simulink model "Pix_FCC_flash"  (R2019b)
settings: Solver=FixedStepAuto  StartTime=0.0  StopTime=inf  RelTol=1e-3  EnableMultiTasking=on
undefined symbols (not defined in the file or in its folder): dev, FCC_PIX_Data, Main, pwm_output0
libraries: px4lib x14, simulink x10, px4Sensorslib x3
(part 1 of 2)
settings Model: ExtModeTrigDuration=10  Creator=The MathWorks, Inc.  LastModifiedBy=guy-m
settings SolverCC: PositivePriorityOrder=on  AutoInsertRateTranBlk=on
settings OptimizationCC: EnhancedBackFolding=on  PassReuseOutputArgsAs=Individual arguments  MaxStackSize=64  OptimizeBlockOrder=speed  DifferentSizesBufferReuse=on  OptimizationCustomize=off  EfficientTunableParamExpr=on
settings DebuggingCC: InheritedTsInSrcMsg=none  MultiTaskCondExecSysMsg=warning  ParameterTunabilityLossMsg=error
settings HardwareCC: ProdBitPerPointer=32  ProdBitPerSizeT=32  ProdBitPerPtrDiffT=32  ProdLargestAtomicInteger=Long  ProdLargestAtomicFloat=Double  ProdWordSize=32  ProdLongLongMode=on  ProdHWDeviceType=ARM Compatible->ARM Cortex
settings SFSimCC: MATLABDynamicMemAlloc=off  CustomCodeUndefinedFunction=UseInterfaceOnly
settings RTWCC: SystemTargetFile=ert.tlc  HardwareBoard=PX4 Pixhawk Series  TLCOptions="-aInlineSetEventsForThisBaseRateFcn=TLC_FALSE -aSuppressMultiTaskScheduler=TLC_FALSE  -aRateBasedStepFcn=0"  TemplateMakefile=ert_default_tmf  Toolchain=GNU Tools for PX4 Autopilots  IncludeHyperlinkInReport=on  TargetLang=C++
settings CodeAppCC: ForceParamTrailComments=on  IgnoreCustomStorageClasses=off  OperatorAnnotations=on  SimulinkDataObjDesc=on  SFDataObjDesc=on  InsertBlockDesc=on
settings ERTTargetCC: SupportVariableSizeSignals=on

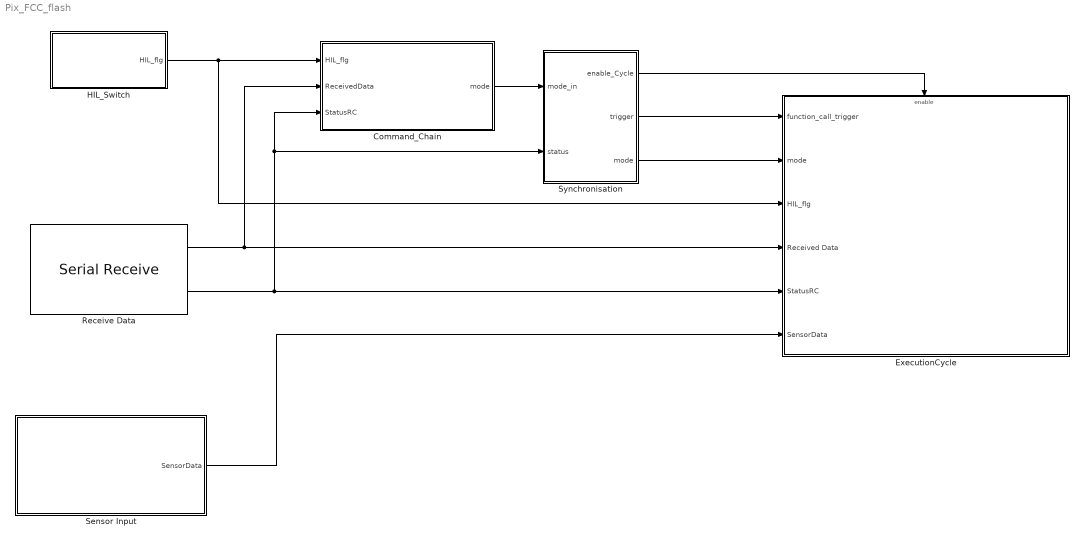
== system Pix_FCC_flash ==
  Command_Chain : Subsystem
  ExecutionCycle : Subsystem
  HIL_Switch : Subsystem
  Receive Data : px4lib/Serial Receive  SCIModule=/dev/ttyS6  DataType=uint8  DataLength=128  OutputStatus=on  SampleTime=0.01  BlockingMode=off  PartialData=off  Timeout=5
      settings: SourceProductName=Embedded Coder Support Package for PX4 Autopilots  SourceProductBaseCode=PX4AUTOPILOTS
  Sensor Input : Subsystem
  Synchronisation : Subsystem
  wires:
  HIL_Switch/1(HIL_flg) -> ExecutionCycle/3(HIL_flg), Command_Chain/1(HIL_flg)
  Command_Chain/1(mode) -> Synchronisation/1(mode_in)
  Synchronisation/1(enable_Cycle) -> ExecutionCycle/Enable
  Synchronisation/2(trigger) -> ExecutionCycle/1(function_call_trigger)
  Receive Data/2 -> ExecutionCycle/5(StatusRC), Command_Chain/3(StatusRC), Synchronisation/2(status)
  Receive Data/1 -> ExecutionCycle/4(Received Data), Command_Chain/2(ReceivedData)
  Synchronisation/3(mode) -> ExecutionCycle/2(mode)
  Sensor Input/1(SensorData) -> ExecutionCycle/6(SensorData)

== system Pix_FCC_flash/Command_Chain ==
  note: sets mode for execution
  note: checks serial input for messages under special command header
  HIL_flg : Inport
  ReceivedData : Inport  Port=2
  StatusRC : Inport  Port=3
  DecodeCommand : Subsystem
  NOT : Logic  Operator=NOT  IconShape=distinctive  AllPortsSameDT=off  OutDataTypeStr=boolean
  SetMode : MATLAB Function  TreatAsAtomicUnit=on
  memory : Subsystem
  mode : Outport  VectorParamsAs1DForOutWhenUnconnected=off
  wires:
  StatusRC/1 -> NOT/1
  ReceivedData/1 -> DecodeCommand/1(message)
  NOT/1 -> DecodeCommand/Enable
  DecodeCommand/2(cmd) -> memory/1(update)
  DecodeCommand/1(cmd_found_flg) -> memory/Enable
  memory/1(standing_cmd) -> SetMode/1(cmd)
  HIL_flg/1 -> SetMode/2(HIL_flg)
  SetMode/1(mode) -> mode/1

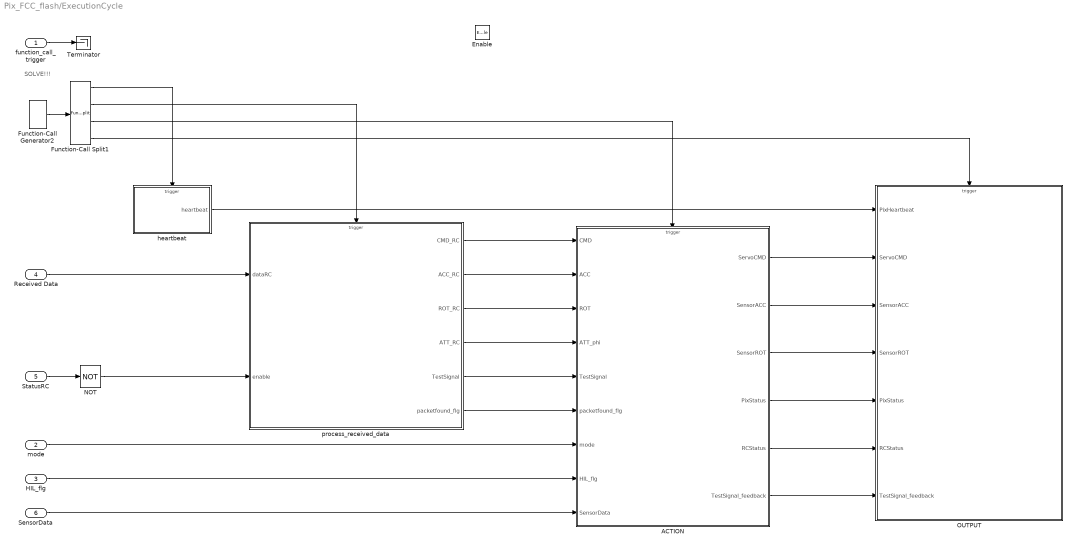
== system Pix_FCC_flash/ExecutionCycle ==
  note: SOLVE!!!
  function_call_trigger : Inport
  mode : Inport  Port=2
  HIL_flg : Inport  Port=3
  Received Data : Inport  Port=4
  StatusRC : Inport  Port=5
  SensorData : Inport  Port=6
  Enable : EnablePort  PropagateVarSize=During execution
  ACTION : Subsystem
  Function-Call Generator2 : simulink/Ports & Subsystems/Function-Call Generator  sample_time=0.01  numberOfIterations=1
  Function-Call Split1 : FunctionCallSplit  IconShape=distinctive  NumOutputPorts=4  OutputPortLayout=default
  NOT : Logic  Operator=NOT  IconShape=distinctive  AllPortsSameDT=off  OutDataTypeStr=boolean
  OUTPUT : Subsystem
  Terminator : Terminator
  heartbeat : Subsystem
  process_received_data : Subsystem
  wires:
  StatusRC/1 -> NOT/1
  NOT/1 -> process_received_data/2(enable)
  Received Data/1 -> process_received_data/1(dataRC)
  process_received_data/1(CMD_RC) -> ACTION/1(CMD)
  process_received_data/2(ACC_RC) -> ACTION/2(ACC)
  process_received_data/3(ROT_RC) -> ACTION/3(ROT)
  process_received_data/4(ATT_RC) -> ACTION/4(ATT_phi)
  process_received_data/6(packetfound_flg) -> ACTION/6(packetfound_flg)
  ACTION/1(ServoCMD) -> OUTPUT/2(ServoCMD)
  ACTION/2(SensorACC) -> OUTPUT/3(SensorACC)
  ACTION/3(SensorROT) -> OUTPUT/4(SensorROT)
  ACTION/4(PixStatus) -> OUTPUT/5(PixStatus)
  heartbeat/1(heartbeat) -> OUTPUT/1(PixHeartbeat)
  Function-Call Split1/1 -> heartbeat/Trigger
  Function-Call Split1/2 -> process_received_data/Trigger
  Function-Call Split1/3 -> ACTION/Trigger
  Function-Call Split1/4 -> OUTPUT/Trigger
  mode/1 -> ACTION/7(mode)
  HIL_flg/1 -> ACTION/8(HIL_flg)
  SensorData/1 -> ACTION/9(SensorData)
  ACTION/5(RCStatus) -> OUTPUT/6(RCStatus)
  process_received_data/5(TestSignal) -> ACTION/5(TestSignal)
  ACTION/6(TestSignal_feedback) -> OUTPUT/7(TestSignal_feedback)
  Function-Call Generator2/1 -> Function-Call Split1/1
  function_call_trigger/1 -> Terminator/1

== system Pix_FCC_flash/HIL_Switch ==
  note: maybe add additional safety? (e.g. for more than one cycle to change?)
  note: in real system this will be done by checking the ADC input for high (HIL connectur plugged in) -> see documentation!!
  Constant : Constant  OutDataTypeStr=boolean
  PX4 Analog Input : px4lib/PX4 Analog Input  Commented=on  sampleTime=0.001
      settings: SourceProductName=Embedded Coder Support Package for PX4 Autopilots  SourceProductBaseCode=PX4AUTOPILOTS
  HIL_flg : Outport  VectorParamsAs1DForOutWhenUnconnected=off
  wires:
  Constant/1 -> HIL_flg/1

== system Pix_FCC_flash/Sensor Input ==
  Accelerometer : px4Sensorslib/Accelerometer  uorbTimeStamp=off  BlockingMode=off  BlockTimeout=1e-3  sampleTime=1/250
      settings: SourceProductName=Embedded Coder Support Package for PX4 Autopilots
  Gyroscope : px4Sensorslib/Gyroscope  uorbTimeStamp=off  BlockingMode=off  BlockTimeout=1e-3  sampleTime=1/250
      settings: SourceProductName=Embedded Coder Support Package for PX4 Autopilots
  Mux : Mux  Inputs=3
  Mux1 : Mux  Inputs=3
  Mux2 : Mux  Inputs=2
  Terminator : Terminator
  Terminator1 : Terminator
  Vehicle Attitude : px4Sensorslib/Vehicle Attitude  rollRate=on  pitchRate=on  yawRate=on  quaternion=on  uorbTimeStamp=off  BlockingMode=off  BlockTimeout=0.001  sampleTime=1/250
      settings: SourceProductName=Embedded Coder Support Package for PX4 Autopilots
  SensorData : Outport  VectorParamsAs1DForOutWhenUnconnected=off
  wires:
  Mux/1 -> Mux2/1
  Mux1/1 -> Mux2/2
  Gyroscope/2 -> Mux1/1
  Accelerometer/1 -> Terminator/1
  Gyroscope/4 -> Mux1/3
  Gyroscope/3 -> Mux1/2
  Accelerometer/3 -> Mux/2
  Accelerometer/4 -> Mux/3
  Accelerometer/2 -> Mux/1
  Gyroscope/1 -> Terminator1/1
  Mux2/1 -> SensorData/1

== system Pix_FCC_flash/Synchronisation ==
  note: SOLVE!!!!
  note: controls the execution of the execution cycle and thereby synchronizes the execution
  mode_in : Inport
  status : Inport  Port=2
  Constant : Constant  Value=0
  ControlExecution : MATLAB Function  TreatAsAtomicUnit=on
  NOT : Logic  Operator=NOT  IconShape=distinctive  AllPortsSameDT=off  OutDataTypeStr=boolean
  trigger_100Hz : Subsystem  Commented=on
  trigger_10Hz : Subsystem  Commented=on
  trigger_inherited : Subsystem  Commented=on
  enable_Cycle : Outport  VectorParamsAs1DForOutWhenUnconnected=off
  trigger : Outport  Port=2  VectorParamsAs1DForOutWhenUnconnected=off
  mode : Outport  Port=3  VectorParamsAs1DForOutWhenUnconnected=off
  wires:
  status/1 -> NOT/1
  mode_in/1 -> mode/1, ControlExecution/1(mode)
  NOT/1 -> ControlExecution/2(status)
  ControlExecution/1(enable_execution) -> enable_Cycle/1
  ControlExecution/2(enable_trigger_inh) -> trigger_inherited/Enable
  ControlExecution/3(enable_trigger_10Hz) -> trigger_10Hz/Enable
  ControlExecution/4(enable_trigger_100Hz) -> trigger_100Hz/Enable
  trigger_inherited/1(trigger) -> ?
  trigger_100Hz/1(trigger) -> ?
  trigger_10Hz/1(trigger) -> ?
  Constant/1 -> trigger/1

== system Pix_FCC_flash/Command_Chain/DecodeCommand ==
  message : Inport
  Enable : EnablePort  PropagateVarSize=During execution
  ConfirmCommand : Subsystem
  DecodeCommand : MATLAB Function  TreatAsAtomicUnit=on
  cmd_found_flg : Outport  VectorParamsAs1DForOutWhenUnconnected=off
  cmd : Outport  Port=2  VectorParamsAs1DForOutWhenUnconnected=off
  wires:
  message/1 -> DecodeCommand/1(message)
  DecodeCommand/2(cmd_found_flg) -> ConfirmCommand/Enable, cmd_found_flg/1
  DecodeCommand/1(cmd) -> ConfirmCommand/1(cmd_received), cmd/1

== system Pix_FCC_flash/Command_Chain/memory ==
  update : Inport
  Enable : EnablePort  PropagateVarSize=During execution
  standing_cmd : Outport  VectorParamsAs1DForOutWhenUnconnected=off
  wires:
  update/1 -> standing_cmd/1

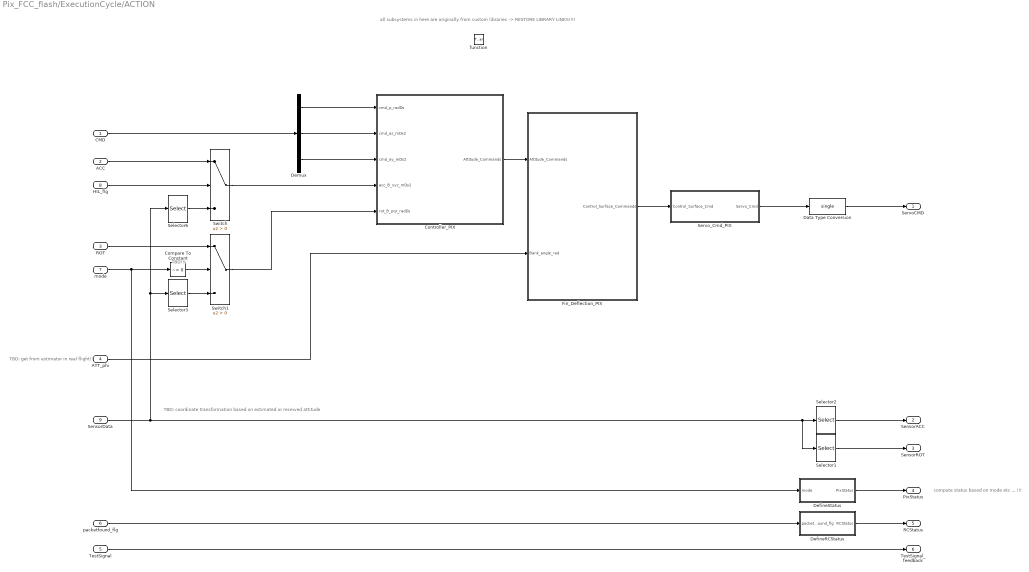
== system Pix_FCC_flash/ExecutionCycle/ACTION ==
  note: TBD: coordinate transformation based on estimated or received attitude
  note: TBD: get from estimator in real flight!!
  note: TBD!!!
  note: compute status based on mode etc ... !!!
  note: all subsystems in here are originally from custom libraries -> RESTORE LIBRARY LINKS!!!!
  CMD : Inport
  ACC : Inport  Port=2
  ROT : Inport  Port=3
  ATT_phi : Inport  Port=4
  TestSignal : Inport  Port=5
  packetfound_flg : Inport  Port=6
  mode : Inport  Port=7
  HIL_flg : Inport  Port=8
  SensorData : Inport  Port=9
  function : TriggerPort  TriggerType=function-call  VariantControl=Variant
  Compare To Constant : simulink/Logic and Bit Operations/Compare To Constant  relop=~=  const=0  OutDataTypeStr=boolean
  Controller_PIX : Subsystem
  Data Type Conversion : DataTypeConversion  OutDataTypeStr=single
  DefineRCStatus : MATLAB Function  TreatAsAtomicUnit=on
  DefineStatus : MATLAB Function  TreatAsAtomicUnit=on
  Demux : Demux  Outputs=3
  Fin_Deflection_PIX : Subsystem
  Selector1 : Selector  InputPortWidth=6  IndexOptions=Index vector (dialog)  Indices=[4,5,6]  OutputSizes=1
  Selector2 : Selector  InputPortWidth=6  IndexOptions=Index vector (dialog)  Indices=[1,2,3]  OutputSizes=1
  Selector3 : Selector  InputPortWidth=6  IndexOptions=Index vector (dialog)  Indices=[4,5,6]  OutputSizes=1
  Selector6 : Selector  InputPortWidth=6  IndexOptions=Index vector (dialog)  Indices=[1,2,3]  OutputSizes=1
  Servo_Cmd_PIX : Subsystem
  Switch : Switch  Criteria=u2 > Threshold
  Switch1 : Switch  Criteria=u2 > Threshold
  ServoCMD : Outport  VectorParamsAs1DForOutWhenUnconnected=off
  SensorACC : Outport  Port=2  VectorParamsAs1DForOutWhenUnconnected=off
  SensorROT : Outport  Port=3  VectorParamsAs1DForOutWhenUnconnected=off
  PixStatus : Outport  Port=4  VectorParamsAs1DForOutWhenUnconnected=off
  RCStatus : Outport  Port=5  VectorParamsAs1DForOutWhenUnconnected=off
  TestSignal_feedback : Outport  Port=6  VectorParamsAs1DForOutWhenUnconnected=off
  wires:
  CMD/1 -> Demux/1
  Servo_Cmd_PIX/1(Servo_Cmd) -> Data Type Conversion/1
  ATT_phi/1 -> Fin_Deflection_PIX/2(Bank_angle_rad)
  Controller_PIX/1(Attitude_Commands) -> Fin_Deflection_PIX/1(Attitude_Commands)
  Fin_Deflection_PIX/1(Control_Surface_Commands) -> Servo_Cmd_PIX/1(Control_Surface_Cmd)
  HIL_flg/1 -> Switch/2
  Switch/1 -> Controller_PIX/4(acc_B_xyz_mDs2)
  Demux/3 -> Controller_PIX/3(cmd_ay_mDs2)
  Demux/2 -> Controller_PIX/2(cmd_az_mDs2)
  Demux/1 -> Controller_PIX/1(cmd_p_radDs)
  Selector2/1 -> SensorACC/1
  Selector1/1 -> SensorROT/1
  ACC/1 -> Switch/1
  Selector6/1 -> Switch/3
  SensorData/1 -> Selector1/1, Selector2/1, Selector3/1, Selector6/1
  Compare To Constant/1 -> Switch1/2
  mode/1 -> DefineStatus/1(mode), Compare To Constant/1
  ROT/1 -> Switch1/1
  Selector3/1 -> Switch1/3
  Switch1/1 -> Controller_PIX/5(rot_B_pqr_radDs)
  packetfound_flg/1 -> DefineRCStatus/1(packetfound_flg)
  DefineStatus/1(PixStatus) -> PixStatus/1
  DefineRCStatus/1(RCStatus) -> RCStatus/1
  TestSignal/1 -> TestSignal_feedback/1
  Data Type Conversion/1 -> ServoCMD/1

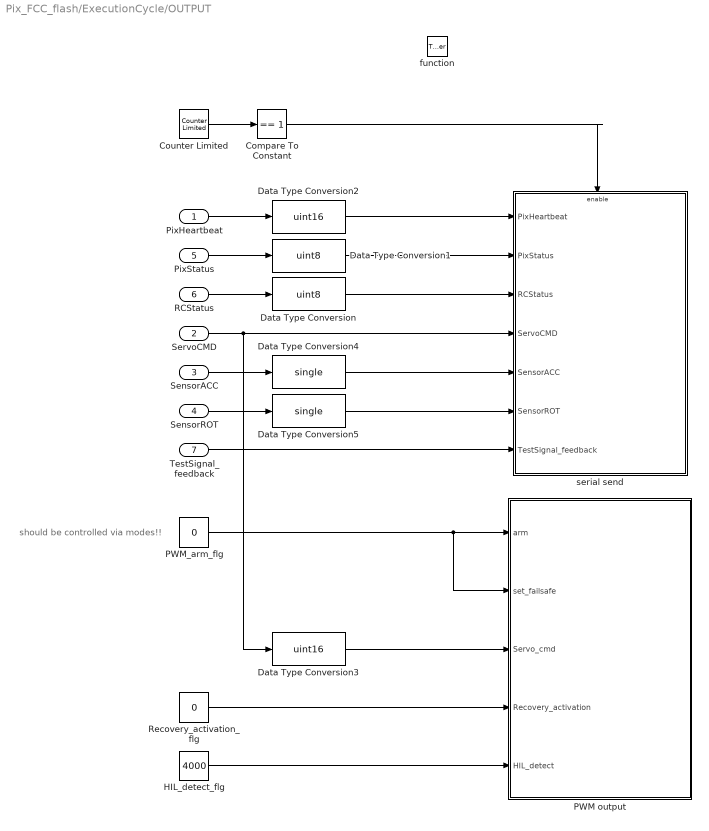
== system Pix_FCC_flash/ExecutionCycle/OUTPUT ==
  note: should be controlled via modes!!
  PixHeartbeat : Inport
  ServoCMD : Inport  Port=2
  SensorACC : Inport  Port=3
  SensorROT : Inport  Port=4
  PixStatus : Inport  Port=5
  RCStatus : Inport  Port=6
  TestSignal_feedback : Inport  Port=7
  function : TriggerPort  TriggerType=function-call  VariantControl=Variant
  Compare To Constant : simulink/Logic and Bit Operations/Compare To Constant  relop===  const=1  OutDataTypeStr=boolean
  Counter Limited : simulink/Sources/Counter Limited  uplimit=1  tsamp=-1
  Data Type Conversion : DataTypeConversion  OutDataTypeStr=uint8
  Data Type Conversion1 : DataTypeConversion  OutDataTypeStr=uint8
  Data Type Conversion2 : DataTypeConversion  OutDataTypeStr=uint16
  Data Type Conversion3 : DataTypeConversion  OutDataTypeStr=uint16
  Data Type Conversion4 : DataTypeConversion  OutDataTypeStr=single
  Data Type Conversion5 : DataTypeConversion  OutDataTypeStr=single
  HIL_detect_flg : Constant  Value=4000  OutDataTypeStr=uint16
  PWM output : Subsystem
  PWM_arm_flg : Constant  Value=0  OutDataTypeStr=boolean
  Recovery_activation_flg : Constant  Value=0  OutDataTypeStr=uint16
  serial send : Subsystem
  wires:
  Counter Limited/1 -> Compare To Constant/1
  Compare To Constant/1 -> serial send/Enable
  PixHeartbeat/1 -> Data Type Conversion2/1
  PixStatus/1 -> Data Type Conversion1/1
  RCStatus/1 -> Data Type Conversion/1
  SensorACC/1 -> Data Type Conversion4/1
  SensorROT/1 -> Data Type Conversion5/1
  Data Type Conversion/1 -> serial send/3(RCStatus)
  Data Type Conversion1/1 -> serial send/2(PixStatus)
  Data Type Conversion2/1 -> serial send/1(PixHeartbeat)
  PWM_arm_flg/1 -> PWM output/2(set_failsafe), PWM output/1(arm)
  HIL_detect_flg/1 -> PWM output/5(HIL_detect)
  Recovery_activation_flg/1 -> PWM output/4(Recovery_activation)
  TestSignal_feedback/1 -> serial send/7(TestSignal_feedback)
  ServoCMD/1 -> serial send/4(ServoCMD), Data Type Conversion3/1
  Data Type Conversion3/1 -> PWM output/3(Servo_cmd)
  Data Type Conversion5/1 -> serial send/6(SensorROT)
  Data Type Conversion4/1 -> serial send/5(SensorACC)

== system Pix_FCC_flash/ExecutionCycle/heartbeat ==
  function : TriggerPort  TriggerType=function-call  VariantControl=Variant
  Add : Sum  Commented=on
  Constant : Constant  Commented=on
  Counter Free-Running : simulink/Sources/Counter Free-Running  NumBits=16  tsamp=-1
  Data Type Conversion1 : DataTypeConversion  Commented=on  OutDataTypeStr=single
  IC : InitialCondition  Commented=on  Value=0
  Memory : Memory  Commented=on  InheritSampleTime=on
  heartbeat : Outport  VectorParamsAs1DForOutWhenUnconnected=off
  wires:
  IC/1 -> Add/2
  Constant/1 -> Add/1
  Add/1 -> Data Type Conversion1/1, Memory/1
  Memory/1 -> IC/1
  Counter Free-Running/1 -> heartbeat/1

== system Pix_FCC_flash/ExecutionCycle/process_received_data ==
  dataRC : Inport
  enable : Inport  Port=2
  function : TriggerPort  TriggerType=function-call  VariantControl=Variant
  Terminator : Terminator
  Terminator1 : Terminator
  Terminator2 : Terminator
  input_hold : Subsystem
  CMD_RC : Outport  VectorParamsAs1DForOutWhenUnconnected=off
  ACC_RC : Outport  Port=2  VectorParamsAs1DForOutWhenUnconnected=off
  ROT_RC : Outport  Port=3  VectorParamsAs1DForOutWhenUnconnected=off
  ATT_RC : Outport  Port=4  VectorParamsAs1DForOutWhenUnconnected=off
  TestSignal : Outport  Port=5  VectorParamsAs1DForOutWhenUnconnected=off
  packetfound_flg : Outport  Port=6  VectorParamsAs1DForOutWhenUnconnected=off
  wires:
  dataRC/1 -> input_hold/1(dataRC)
  input_hold/9(packetfound_flg) -> packetfound_flg/1
  enable/1 -> input_hold/Enable
  input_hold/2(SimStatus) -> Terminator/1
  input_hold/3(SimRCStatus) -> Terminator1/1
  input_hold/1(SimHeartbeat) -> Terminator2/1
  input_hold/4(CMD) -> CMD_RC/1
  input_hold/5(ACC) -> ACC_RC/1
  input_hold/6(ROT) -> ROT_RC/1
  input_hold/7(ATT) -> ATT_RC/1
  input_hold/8(TestSignal) -> TestSignal/1

== system Pix_FCC_flash/Synchronisation/trigger_100Hz ==
  Enable : EnablePort
  Function-Call Generator2 : simulink/Ports & Subsystems/Function-Call Generator  sample_time=0.01  numberOfIterations=1
  trigger : Outport  VectorParamsAs1DForOutWhenUnconnected=off
  wires:
  Function-Call Generator2/1 -> trigger/1

== system Pix_FCC_flash/Synchronisation/trigger_10Hz ==
  Enable : EnablePort
  Function-Call Generator2 : simulink/Ports & Subsystems/Function-Call Generator  sample_time=0.1  numberOfIterations=1
  trigger : Outport  VectorParamsAs1DForOutWhenUnconnected=off
  wires:
  Function-Call Generator2/1 -> trigger/1

== system Pix_FCC_flash/Synchronisation/trigger_inherited ==
  Enable : EnablePort
  Function-Call Generator2 : simulink/Ports & Subsystems/Function-Call Generator  sample_time=-1  numberOfIterations=1
  trigger : Outport  VectorParamsAs1DForOutWhenUnconnected=off
  wires:
  Function-Call Generator2/1 -> trigger/1

== system Pix_FCC_flash/Command_Chain/DecodeCommand/ConfirmCommand ==
  cmd_received : Inport
  Enable : EnablePort  PropagateVarSize=During execution
  Function-Call Generator1 : simulink/Ports & Subsystems/Function-Call Generator  sample_time=-1  numberOfIterations=1
  Function-Call Split : FunctionCallSplit  IconShape=distinctive  NumOutputPorts=6  OutputPortLayout=default
  Send Data : Subsystem
  Send Header : Subsystem  TreatAsAtomicUnit=on
  Send RC Confrimation : Subsystem  TreatAsAtomicUnit=on
  Send Terminator : Subsystem  TreatAsAtomicUnit=on
  Send WhiteNoise Beginning : Subsystem  TreatAsAtomicUnit=on
  Send WhiteNoise End : Subsystem  TreatAsAtomicUnit=on
  pack : MATLAB Function  TreatAsAtomicUnit=on
  wires:
  Function-Call Split/6 -> Send WhiteNoise End/Trigger
  Function-Call Split/5 -> Send Terminator/Trigger
  Function-Call Split/4 -> Send Data/Trigger
  Function-Call Split/1 -> Send WhiteNoise Beginning/Trigger
  pack/1(send) -> Send Data/1(data)
  Function-Call Generator1/1 -> Function-Call Split/1
  Function-Call Split/2 -> Send Header/Trigger
  Function-Call Split/3 -> Send RC Confrimation/Trigger
  cmd_received/1 -> pack/1(in)

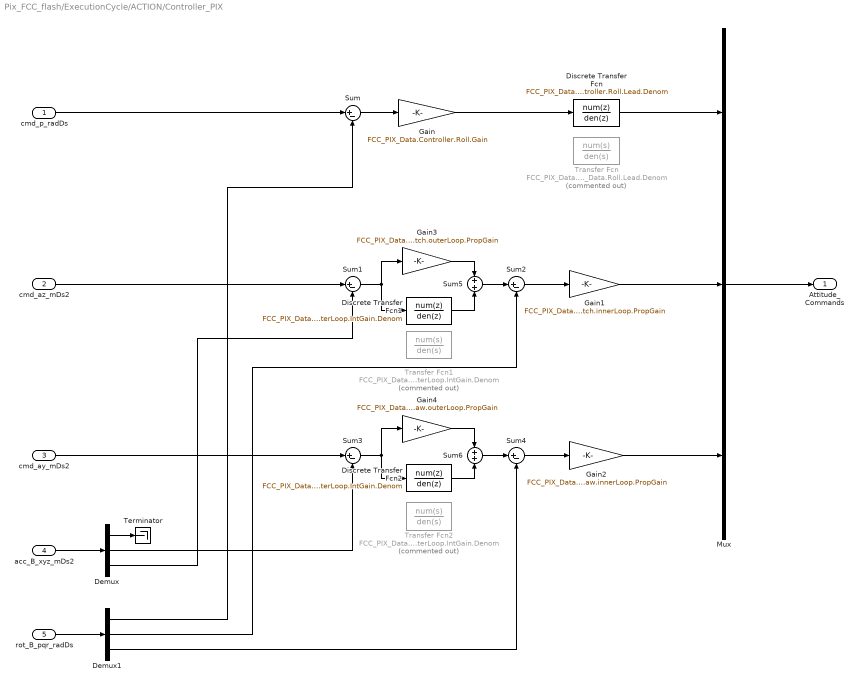
== system Pix_FCC_flash/ExecutionCycle/ACTION/Controller_PIX ==
  cmd_p_radDs : Inport
  cmd_az_mDs2 : Inport  Port=2
  cmd_ay_mDs2 : Inport  Port=3
  acc_B_xyz_mDs2 : Inport  Port=4
  rot_B_pqr_radDs : Inport  Port=5
  Demux : Demux  Outputs=3
  Demux1 : Demux  Outputs=3
  Discrete Transfer Fcn : DiscreteTransferFcn  Numerator=FCC_PIX_Data.Controller.Roll.Lead.Num  Denominator=FCC_PIX_Data.Controller.Roll.Lead.Denom
  Discrete Transfer Fcn1 : DiscreteTransferFcn  Numerator=FCC_PIX_Data.Controller.Pitch.outerLoop.IntGain.Num  Denominator=FCC_PIX_Data.Controller.Pitch.outerLoop.IntGain.Denom
  Discrete Transfer Fcn2 : DiscreteTransferFcn  Numerator=FCC_PIX_Data.Controller.Yaw.outerLoop.IntGain.Num  Denominator=FCC_PIX_Data.Controller.Yaw.outerLoop.IntGain.Denom
  Gain : Gain  Gain=FCC_PIX_Data.Controller.Roll.Gain
  Gain1 : Gain  Gain=FCC_PIX_Data.Controller.Pitch.innerLoop.PropGain
  Gain2 : Gain  Gain=FCC_PIX_Data.Controller.Yaw.innerLoop.PropGain
  Gain3 : Gain  Gain=FCC_PIX_Data.Controller.Pitch.outerLoop.PropGain
  Gain4 : Gain  Gain=FCC_PIX_Data.Controller.Yaw.outerLoop.PropGain
  Mux : Mux  Inputs=3
  Sum{,1..4} (5 alike) : Sum  Inputs=|+-
  Sum5 : Sum  Inputs=+|+
  Sum6 : Sum  Inputs=+|+
  Terminator : Terminator
  Transfer Fcn : TransferFcn  Commented=on  Numerator=FCC_PIX_Data.Roll.Lead.Num  Denominator=FCC_PIX_Data.Roll.Lead.Denom
  Transfer Fcn1 : TransferFcn  Commented=on  Numerator=FCC_PIX_Data.Controller.Pitch.outerLoop.IntGain.Num  Denominator=FCC_PIX_Data.Controller.Pitch.outerLoop.IntGain.Denom
  Transfer Fcn2 : TransferFcn  Commented=on  Numerator=FCC_PIX_Data.Controller.Yaw.outerLoop.IntGain.Num  Denominator=FCC_PIX_Data.Controller.Yaw.outerLoop.IntGain.Denom
  Attitude_Commands : Outport  VectorParamsAs1DForOutWhenUnconnected=off
  wires:
  Demux/1 -> Terminator/1
  Demux/3 -> Sum1/2
  Demux/2 -> Sum3/2
  Demux1/3 -> Sum4/2
  Demux1/2 -> Sum2/2
  Demux1/1 -> Sum/2
  rot_B_pqr_radDs/1 -> Demux1/1
  acc_B_xyz_mDs2/1 -> Demux/1
  Mux/1 -> Attitude_Commands/1
  Discrete Transfer Fcn/1 -> Mux/1
  Gain1/1 -> Mux/2
  Gain2/1 -> Mux/3
  cmd_az_mDs2/1 -> Sum1/1
  cmd_ay_mDs2/1 -> Sum3/1
  cmd_p_radDs/1 -> Sum/1
  Sum3/1 -> Discrete Transfer Fcn2/1, Gain4/1
  Discrete Transfer Fcn2/1 -> Sum6/2
  Gain4/1 -> Sum6/1
  Sum/1 -> Gain/1
  Sum4/1 -> Gain2/1
  Sum2/1 -> Gain1/1
  Gain/1 -> Discrete Transfer Fcn/1
  Sum5/1 -> Sum2/1
  Discrete Transfer Fcn1/1 -> Sum5/2
  Gain3/1 -> Sum5/1
  Sum1/1 -> Discrete Transfer Fcn1/1, Gain3/1
  Sum6/1 -> Sum4/1

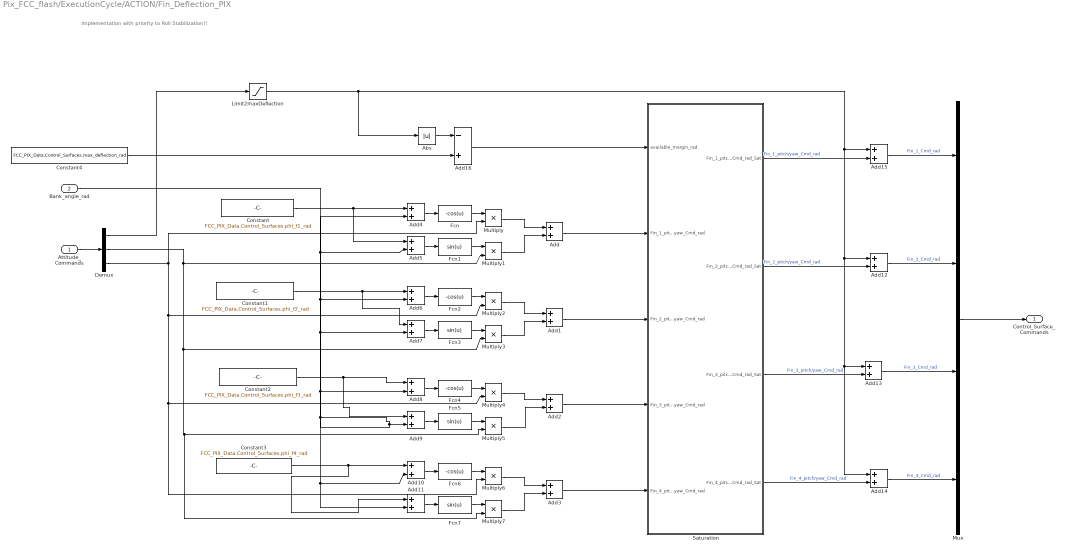
== system Pix_FCC_flash/ExecutionCycle/ACTION/Fin_Deflection_PIX ==
  note: Implementation with priority to Roll Stabilization!!
  Attitude_Commands : Inport
  Bank_angle_rad : Inport  Port=2
  Abs : Abs
  Add{,1..15} (16 alike) : Sum
  Add16 : Sum  Inputs=-+
  Constant : Constant  Value=FCC_PIX_Data.Control_Surfaces.phi_f1_rad
  Constant1 : Constant  Value=FCC_PIX_Data.Control_Surfaces.phi_f2_rad
  Constant2 : Constant  Value=FCC_PIX_Data.Control_Surfaces.phi_f3_rad
  Constant3 : Constant  Value=FCC_PIX_Data.Control_Surfaces.phi_f4_rad
  Constant4 : Constant  Value=FCC_PIX_Data.Control_Surfaces.max_deflection_rad
  Demux : Demux  Outputs=3
  Fcn{,2,4,6} (4 alike) : Fcn  Expr=-cos(u)
  Fcn{1,3,5,7} (4 alike) : Fcn  Expr=sin(u)
  Limit2maxDeflection : Saturate  UpperLimit=FCC_PIX_Data.Control_Surfaces.max_deflection_rad  LowerLimit=-FCC_PIX_Data.Control_Surfaces.max_deflection_rad
  Multiply{,1..7} (8 alike) : Product
  Mux : Mux
  Saturation : Subsystem
  Control_Surface_Commands : Outport  VectorParamsAs1DForOutWhenUnconnected=off
  wires:
  Limit2maxDeflection/1 -> Add15/1, Add12/1, Add13/1, Add14/1, Abs/1
  Saturation/4(Fin_4_pitch/yaw_Cmd_rad_Sat) -> Add14/2  "Fin_4_pitch/yaw_Cmd_rad"
  Saturation/3(Fin_3_pitch/yaw_Cmd_rad_Sat) -> Add13/2  "Fin_3_pitch/yaw_Cmd_rad"
  Saturation/2(Fin_2_pitch/yaw_Cmd_rad_Sat) -> Add12/2  "Fin_2_pitch/yaw_Cmd_rad"
  Saturation/1(Fin_1_pitch/yaw_Cmd_rad_Sat) -> Add15/2  "Fin_1_pitch/yaw_Cmd_rad"
  Add16/1 -> Saturation/1(available_margin_rad)
  Constant4/1 -> Add16/2
  Abs/1 -> Add16/1
  Demux/1 -> Limit2maxDeflection/1
  Add14/1 -> Mux/4  "Fin_4_Cmd_rad"
  Add13/1 -> Mux/3  "Fin_3_Cmd_rad"
  Add12/1 -> Mux/2  "Fin_2_Cmd_rad"
  Add15/1 -> Mux/1  "Fin_1_Cmd_rad"
  Add3/1 -> Saturation/5(Fin_4_pitch/yaw_Cmd_rad)
  Add2/1 -> Saturation/4(Fin_3_pitch/yaw_Cmd_rad)
  Add1/1 -> Saturation/3(Fin_2_pitch/yaw_Cmd_rad)
  Add/1 -> Saturation/2(Fin_1_pitch/yaw_Cmd_rad)
  Mux/1 -> Control_Surface_Commands/1
  Attitude_Commands/1 -> Demux/1
  Constant/1 -> Add4/1, Add5/1
  Constant1/1 -> Add6/1, Add7/1
  Constant2/1 -> Add8/1, Add9/1
  Constant3/1 -> Add10/1, Add11/1
  Bank_angle_rad/1 -> Add9/2, Add8/2, Add6/2, Add5/2, Add4/2, Add7/2, Add10/2, Add11/2
  Multiply7/1 -> Add3/2
  Multiply6/1 -> Add3/1
  Multiply5/1 -> Add2/2
  Multiply4/1 -> Add2/1
  Multiply3/1 -> Add1/2
  Multiply2/1 -> Add1/1
  Multiply1/1 -> Add/2
  Multiply/1 -> Add/1
  Demux/3 -> Multiply2/2, Multiply4/2, Multiply6/2, Multiply/2
  Demux/2 -> Multiply1/2, Multiply3/2, Multiply7/2, Multiply5/2
  Fcn7/1 -> Multiply7/1
  Add10/1 -> Fcn6/1
  Fcn6/1 -> Multiply6/1
  Add11/1 -> Fcn7/1
  Add9/1 -> Fcn5/1
  Fcn4/1 -> Multiply4/1
  Add8/1 -> Fcn4/1
  Fcn5/1 -> Multiply5/1
  Fcn3/1 -> Multiply3/1
  Fcn2/1 -> Multiply2/1
  Add6/1 -> Fcn2/1
  Add7/1 -> Fcn3/1
  Fcn1/1 -> Multiply1/1
  Add5/1 -> Fcn1/1
  Fcn/1 -> Multiply/1
  Add4/1 -> Fcn/1

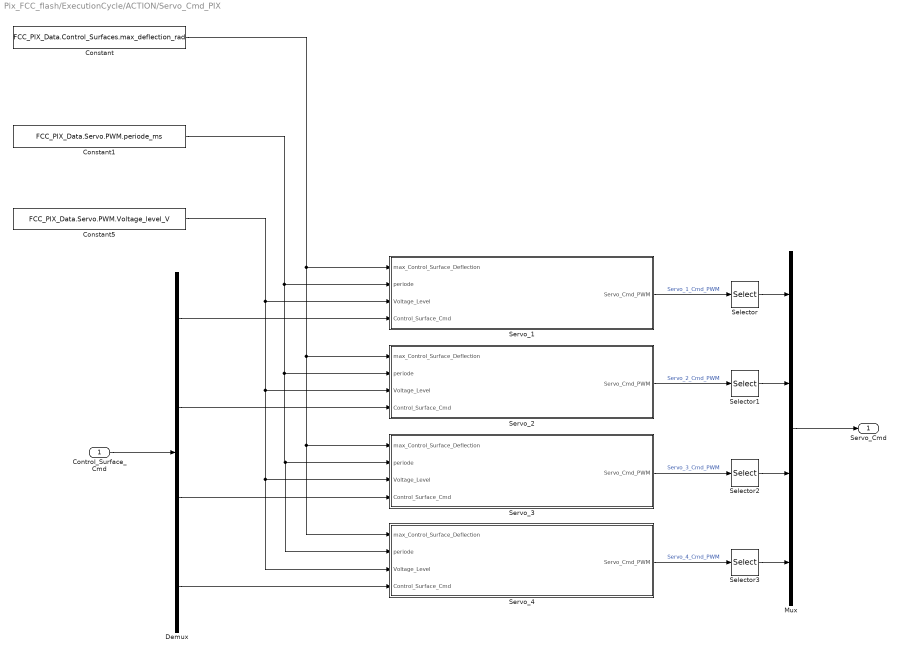
== system Pix_FCC_flash/ExecutionCycle/ACTION/Servo_Cmd_PIX ==
  Control_Surface_Cmd : Inport
  Constant : Constant  Value=FCC_PIX_Data.Control_Surfaces.max_deflection_rad
  Constant1 : Constant  Value=FCC_PIX_Data.Servo.PWM.periode_ms
  Constant5 : Constant  Value=FCC_PIX_Data.Servo.PWM.Voltage_level_V
  Demux : Demux
  Mux : Mux
  Selector{,1..3} (4 alike) : Selector  InputPortWidth=3  IndexOptions=Index vector (dialog)  Indices=[1]  OutputSizes=1
  Servo_1 : Subsystem
  Servo_2 : Subsystem
  Servo_3 : Subsystem
  Servo_4 : Subsystem
  Servo_Cmd : Outport  VectorParamsAs1DForOutWhenUnconnected=off
  wires:
  Selector3/1 -> Mux/4
  Selector2/1 -> Mux/3
  Selector/1 -> Mux/1
  Selector1/1 -> Mux/2
  Demux/1 -> Servo_1/4(Control_Surface_Cmd)
  Demux/2 -> Servo_2/4(Control_Surface_Cmd)
  Demux/3 -> Servo_3/4(Control_Surface_Cmd)
  Demux/4 -> Servo_4/4(Control_Surface_Cmd)
  Servo_4/1(Servo_Cmd_PWM) -> Selector3/1  "Servo_4_Cmd_PWM"
  Servo_3/1(Servo_Cmd_PWM) -> Selector2/1  "Servo_3_Cmd_PWM"
  Servo_2/1(Servo_Cmd_PWM) -> Selector1/1  "Servo_2_Cmd_PWM"
  Constant5/1 -> Servo_1/3(Voltage_Level), Servo_3/3(Voltage_Level), Servo_4/3(Voltage_Level), Servo_2/3(Voltage_Level)
  Constant1/1 -> Servo_1/2(periode), Servo_3/2(periode), Servo_4/2(periode), Servo_2/2(periode)
  Constant/1 -> Servo_1/1(max_Control_Surface_Deflection), Servo_3/1(max_Control_Surface_Deflection), Servo_4/1(max_Control_Surface_Deflection), Servo_2/1(max_Control_Surface_Deflection)
  Servo_1/1(Servo_Cmd_PWM) -> Selector/1  "Servo_1_Cmd_PWM"
  Mux/1 -> Servo_Cmd/1
  Control_Surface_Cmd/1 -> Demux/1

== system Pix_FCC_flash/ExecutionCycle/OUTPUT/PWM output ==
  arm : Inport
  set_failsafe : Inport  Port=2
  Servo_cmd : Inport  Port=3
  Recovery_activation : Inport  Port=4
  HIL_detect : Inport  Port=5
  Demux : Demux
  PX4 PWM Output : px4lib/PX4 PWM Output  pwmDevice=Main (/dev/pwm_output0)  pwmChannel1_=on  pwmChannel2_=on  pwmChannel3_=on  pwmChannel4_=on  pwmChannel5_=on  pwmChannel6_=on  pwmChannel7_=off  pwmChannel8_=off  forceTerminateFailsafe=off  outputErrorStatus=off
      settings: SourceProductName=Embedded Coder Support Package for PX4 Autopilots  SourceProductBaseCode=PX4AUTOPILOTS
  ms2us_{1..4} (4 alike) : Gain  Gain=1000  OutDataTypeStr=uint16
  wires:
  Demux/1 -> ms2us_1/1
  Demux/3 -> ms2us_3/1
  Demux/4 -> ms2us_4/1
  ms2us_1/1 -> PX4 PWM Output/3
  Recovery_activation/1 -> PX4 PWM Output/7
  ms2us_2/1 -> PX4 PWM Output/4
  Servo_cmd/1 -> Demux/1
  Demux/2 -> ms2us_2/1
  ms2us_4/1 -> PX4 PWM Output/6
  ms2us_3/1 -> PX4 PWM Output/5
  HIL_detect/1 -> PX4 PWM Output/8
  arm/1 -> PX4 PWM Output/1
  set_failsafe/1 -> PX4 PWM Output/2

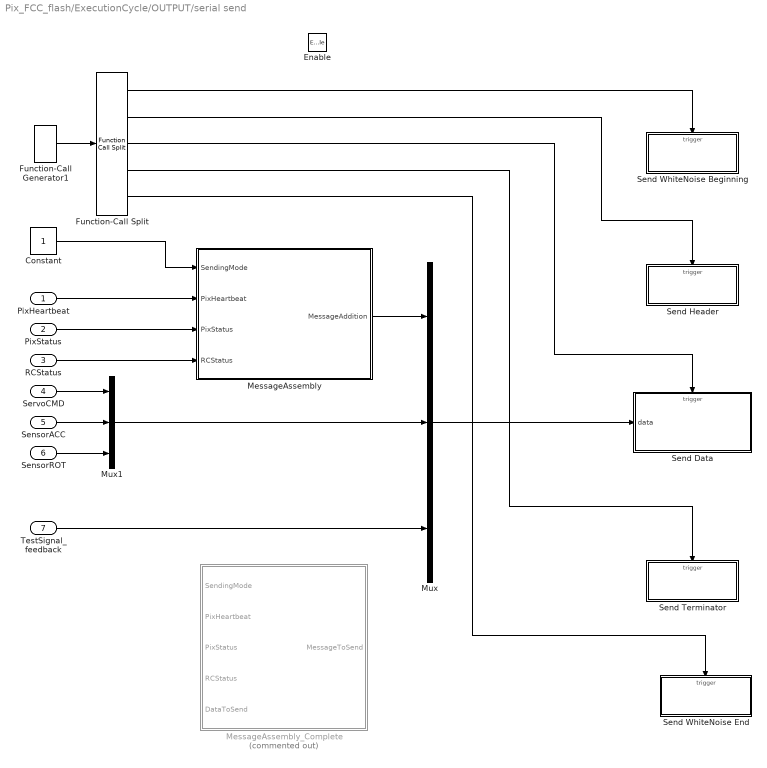
== system Pix_FCC_flash/ExecutionCycle/OUTPUT/serial send ==
  PixHeartbeat : Inport
  PixStatus : Inport  Port=2
  RCStatus : Inport  Port=3
  ServoCMD : Inport  Port=4
  SensorACC : Inport  Port=5
  SensorROT : Inport  Port=6
  TestSignal_feedback : Inport  Port=7
  Enable : EnablePort
  Constant : Constant  OutDataTypeStr=double
  Function-Call Generator1 : simulink/Ports & Subsystems/Function-Call Generator  sample_time=-1  numberOfIterations=1
  Function-Call Split : FunctionCallSplit  IconShape=distinctive  NumOutputPorts=5  OutputPortLayout=default
  MessageAssembly : MATLAB Function  TreatAsAtomicUnit=on
  MessageAssembly_Complete : MATLAB Function  Commented=on  TreatAsAtomicUnit=on
  Mux : Mux  Inputs=3
  Mux1 : Mux  Inputs=3
  Send Data : Subsystem
  Send Header : Subsystem  TreatAsAtomicUnit=on
  Send Terminator : Subsystem  TreatAsAtomicUnit=on
  Send WhiteNoise Beginning : Subsystem  TreatAsAtomicUnit=on
  Send WhiteNoise End : Subsystem  TreatAsAtomicUnit=on
  wires:
  SensorROT/1 -> Mux1/3
  SensorACC/1 -> Mux1/2
  ServoCMD/1 -> Mux1/1
  Constant/1 -> MessageAssembly/1(SendingMode)
  PixHeartbeat/1 -> MessageAssembly/2(PixHeartbeat)
  PixStatus/1 -> MessageAssembly/3(PixStatus)
  RCStatus/1 -> MessageAssembly/4(RCStatus)
  MessageAssembly/1(MessageAddition) -> Mux/1
  Mux1/1 -> Mux/2
  Function-Call Generator1/1 -> Function-Call Split/1
  Mux/1 -> Send Data/1(data)
  Function-Call Split/1 -> Send WhiteNoise Beginning/Trigger
  Function-Call Split/2 -> Send Header/Trigger
  Function-Call Split/3 -> Send Data/Trigger
  Function-Call Split/4 -> Send Terminator/Trigger
  Function-Call Split/5 -> Send WhiteNoise End/Trigger
  TestSignal_feedback/1 -> Mux/3

== system Pix_FCC_flash/ExecutionCycle/process_received_data/input_hold ==
  note: holds last received values if failed to extract message
  dataRC : Inport
  Enable : EnablePort  PropagateVarSize=During execution
  ByteUnpack : MATLAB Function  TreatAsAtomicUnit=on
  ExtractMessage : MATLAB Function  TreatAsAtomicUnit=on
  hold : Subsystem
  SimHeartbeat : Outport  VectorParamsAs1DForOutWhenUnconnected=off
  SimStatus : Outport  Port=2  VectorParamsAs1DForOutWhenUnconnected=off
  SimRCStatus : Outport  Port=3  VectorParamsAs1DForOutWhenUnconnected=off
  CMD : Outport  Port=4  VectorParamsAs1DForOutWhenUnconnected=off
  ACC : Outport  Port=5  VectorParamsAs1DForOutWhenUnconnected=off
  ROT : Outport  Port=6  VectorParamsAs1DForOutWhenUnconnected=off
  ATT : Outport  Port=7  VectorParamsAs1DForOutWhenUnconnected=off
  TestSignal : Outport  Port=8  VectorParamsAs1DForOutWhenUnconnected=off
  packetfound_flg : Outport  Port=9  VectorParamsAs1DForOutWhenUnconnected=off
  wires:
  ExtractMessage/1(message) -> ByteUnpack/1(message)
  dataRC/1 -> ExtractMessage/1(data)
  ExtractMessage/2(packetfound) -> hold/Enable, packetfound_flg/1
  ByteUnpack/2(SimStatus) -> hold/2(SimStatus_update)
  ByteUnpack/3(SimRCStatus) -> hold/3(SimRCStatus_update)
  ByteUnpack/1(SimHeartbeat) -> hold/1(SimHeartbeat_update)
  ByteUnpack/4(CMD) -> hold/4(CMD_update)
  ByteUnpack/5(ACC) -> hold/5(ACC_update)
  ByteUnpack/6(ROT) -> hold/6(ROT_update)
  ByteUnpack/7(ATT) -> hold/7(ATT_update)
  hold/7(ATT) -> ATT/1
  hold/6(ROT) -> ROT/1
  hold/5(ACC) -> ACC/1
  hold/4(CMD) -> CMD/1
  hold/3(SimRCStatus) -> SimRCStatus/1
  hold/2(SimStatus) -> SimStatus/1
  hold/1(SimHeartbeat) -> SimHeartbeat/1
  ByteUnpack/8(TestSignal) -> hold/8(TestSignal_update)
  hold/8(TestSignal) -> TestSignal/1

== system Pix_FCC_flash/Command_Chain/DecodeCommand/ConfirmCommand/Send Data ==
  data : Inport
  function : TriggerPort  TriggerType=function-call  VariantControl=Variant
  Serial Transmit : px4lib/Serial Transmit  SCIModule=/dev/ttyS6
      settings: SourceProductName=Embedded Coder Support Package for PX4 Autopilots  SourceProductBaseCode=PX4AUTOPILOTS
  wires:
  data/1 -> Serial Transmit/1

== system Pix_FCC_flash/Command_Chain/DecodeCommand/ConfirmCommand/Send Header ==
  function : TriggerPort  TriggerType=function-call  VariantControl=Variant
  Header : Constant  Value=[9 9]  OutDataTypeStr=uint8  SampleTime=-1
  Serial Transmit : px4lib/Serial Transmit  SCIModule=/dev/ttyS6
      settings: SourceProductName=Embedded Coder Support Package for PX4 Autopilots  SourceProductBaseCode=PX4AUTOPILOTS
  wires:
  Header/1 -> Serial Transmit/1

== system Pix_FCC_flash/Command_Chain/DecodeCommand/ConfirmCommand/Send RC Confrimation ==
  function : TriggerPort  TriggerType=function-call  VariantControl=Variant
  Header : Constant  Value=[1]  OutDataTypeStr=uint8  SampleTime=-1
  Serial Transmit : px4lib/Serial Transmit  SCIModule=/dev/ttyS6
      settings: SourceProductName=Embedded Coder Support Package for PX4 Autopilots  SourceProductBaseCode=PX4AUTOPILOTS
  wires:
  Header/1 -> Serial Transmit/1

== system Pix_FCC_flash/Command_Chain/DecodeCommand/ConfirmCommand/Send Terminator ==
  function : TriggerPort  TriggerType=function-call  VariantControl=Variant
  Header : Constant  Value=[9 9]  OutDataTypeStr=uint8  SampleTime=-1
  Serial Transmit : px4lib/Serial Transmit  SCIModule=/dev/ttyS6
      settings: SourceProductName=Embedded Coder Support Package for PX4 Autopilots  SourceProductBaseCode=PX4AUTOPILOTS
  wires:
  Header/1 -> Serial Transmit/1

== system Pix_FCC_flash/Command_Chain/DecodeCommand/ConfirmCommand/Send WhiteNoise Beginning ==
  function : TriggerPort  TriggerType=function-call  VariantControl=Variant
  Header : Constant  Value=[0 0 0 0 0]  OutDataTypeStr=uint8  SampleTime=-1
  Serial Transmit : px4lib/Serial Transmit  SCIModule=/dev/ttyS6
      settings: SourceProductName=Embedded Coder Support Package for PX4 Autopilots  SourceProductBaseCode=PX4AUTOPILOTS
  wires:
  Header/1 -> Serial Transmit/1

== system Pix_FCC_flash/Command_Chain/DecodeCommand/ConfirmCommand/Send WhiteNoise End ==
  function : TriggerPort  TriggerType=function-call  VariantControl=Variant
  Header : Constant  Value=[0 0 0 0 0]  OutDataTypeStr=uint8  SampleTime=-1
  Serial Transmit : px4lib/Serial Transmit  SCIModule=/dev/ttyS6
      settings: SourceProductName=Embedded Coder Support Package for PX4 Autopilots  SourceProductBaseCode=PX4AUTOPILOTS
  wires:
  Header/1 -> Serial Transmit/1

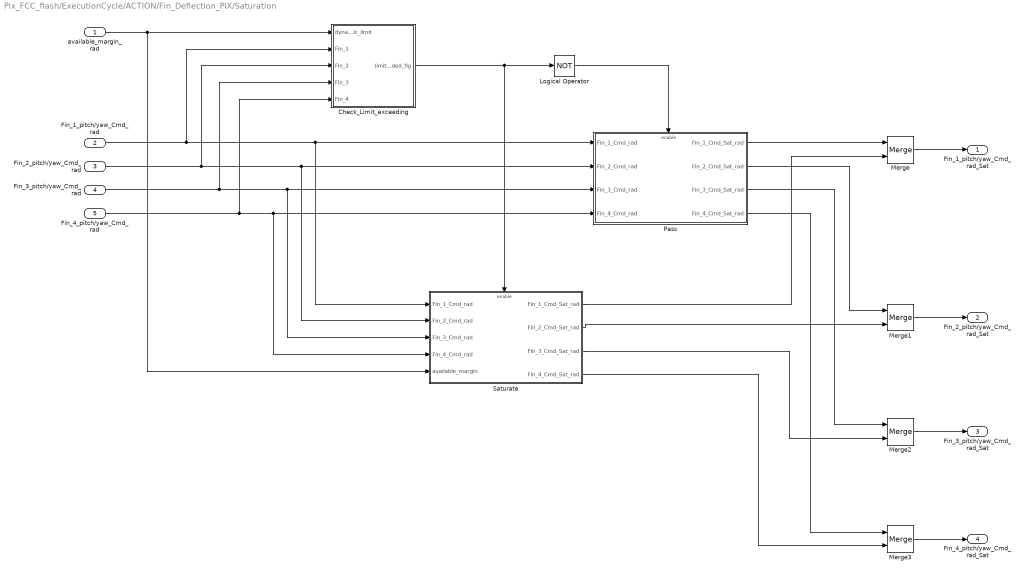
== system Pix_FCC_flash/ExecutionCycle/ACTION/Fin_Deflection_PIX/Saturation ==
  available_margin_rad : Inport
  Fin_1_pitch/yaw_Cmd_rad : Inport  Port=2
  Fin_2_pitch/yaw_Cmd_rad : Inport  Port=3
  Fin_3_pitch/yaw_Cmd_rad : Inport  Port=4
  Fin_4_pitch/yaw_Cmd_rad : Inport  Port=5
  Check_Limit_exceeding : Subsystem
  Logical Operator : Logic  Operator=NOT  AllPortsSameDT=off  OutDataTypeStr=boolean
  Merge{,1..3} (4 alike) : Merge
  Pass : Subsystem
  Saturate : Subsystem
  Fin_1_pitch/yaw_Cmd_rad_Sat : Outport  VectorParamsAs1DForOutWhenUnconnected=off
  Fin_2_pitch/yaw_Cmd_rad_Sat : Outport  Port=2  VectorParamsAs1DForOutWhenUnconnected=off
  Fin_3_pitch/yaw_Cmd_rad_Sat : Outport  Port=3  VectorParamsAs1DForOutWhenUnconnected=off
  Fin_4_pitch/yaw_Cmd_rad_Sat : Outport  Port=4  VectorParamsAs1DForOutWhenUnconnected=off
  wires:
  available_margin_rad/1 -> Check_Limit_exceeding/1(dynamic_limit), Saturate/5(available_margin)
  Saturate/4(Fin_4_Cmd_Sat_rad) -> Merge3/2
  Saturate/3(Fin_3_Cmd_Sat_rad) -> Merge2/2
  Saturate/2(Fin_2_Cmd_Sat_rad) -> Merge1/2
  Saturate/1(Fin_1_Cmd_Sat_rad) -> Merge/2
  Pass/4(Fin_4_Cmd_Sat_rad) -> Merge3/1
  Pass/3(Fin_3_Cmd_Sat_rad) -> Merge2/1
  Pass/2(Fin_2_Cmd_Sat_rad) -> Merge1/1
  Pass/1(Fin_1_Cmd_Sat_rad) -> Merge/1
  Merge2/1 -> Fin_3_pitch/yaw_Cmd_rad_Sat/1
  Logical Operator/1 -> Pass/Enable
  Check_Limit_exceeding/1(limit_exceeded_flg) -> Logical Operator/1, Saturate/Enable
  Merge1/1 -> Fin_2_pitch/yaw_Cmd_rad_Sat/1
  Merge3/1 -> Fin_4_pitch/yaw_Cmd_rad_Sat/1
  Merge/1 -> Fin_1_pitch/yaw_Cmd_rad_Sat/1
  Fin_4_pitch/yaw_Cmd_rad/1 -> Pass/4(Fin_4_Cmd_rad), Saturate/4(Fin_4_Cmd_rad), Check_Limit_exceeding/5(Fin_4)
  Fin_3_pitch/yaw_Cmd_rad/1 -> Saturate/3(Fin_3_Cmd_rad), Pass/3(Fin_3_Cmd_rad), Check_Limit_exceeding/4(Fin_3)
  Fin_2_pitch/yaw_Cmd_rad/1 -> Saturate/2(Fin_2_Cmd_rad), Pass/2(Fin_2_Cmd_rad), Check_Limit_exceeding/3(Fin_2)
  Fin_1_pitch/yaw_Cmd_rad/1 -> Pass/1(Fin_1_Cmd_rad), Saturate/1(Fin_1_Cmd_rad), Check_Limit_exceeding/2(Fin_1)

== system Pix_FCC_flash/ExecutionCycle/ACTION/Servo_Cmd_PIX/Servo_1 ==
  max_Control_Surface_Deflection : Inport
  periode : Inport  Port=2
  Voltage_Level : Inport  Port=3
  Control_Surface_Cmd : Inport  Port=4
  Add : Sum
  Constant2 : Constant  Value=FCC_PIX_Data.Servo.PWM.Pulswidth_cmd_middle_pos_ms
  Constant6 : Constant  Value=FCC_PIX_Data.Servo.PWM.Pulswidth_cmd_max_ms-FCC_PIX_Data.Servo.PWM.Pulswidth_cmd_middle_pos_ms
  Divide : Product  Inputs=*/
  Mux : Mux  Inputs=3
  Product : Product
  Saturation : Saturate  UpperLimit=FCC_PIX_Data.Servo.PWM.Pulswidth_cmd_max_ms  LowerLimit=FCC_PIX_Data.Servo.PWM.Pulswidth_cmd_min_ms
  Servo_Cmd_PWM : Outport  VectorParamsAs1DForOutWhenUnconnected=off
  wires:
  Mux/1 -> Servo_Cmd_PWM/1
  max_Control_Surface_Deflection/1 -> Divide/2
  periode/1 -> Mux/2  "periode_ms"
  Saturation/1 -> Mux/1  "pulse_width_ms"
  Constant6/1 -> Product/1
  Product/1 -> Add/2
  Control_Surface_Cmd/1 -> Divide/1
  Voltage_Level/1 -> Mux/3  "voltage_level_V"
  Add/1 -> Saturation/1
  Divide/1 -> Product/2
  Constant2/1 -> Add/1

== system Pix_FCC_flash/ExecutionCycle/ACTION/Servo_Cmd_PIX/Servo_2 ==
  max_Control_Surface_Deflection : Inport
  periode : Inport  Port=2
  Voltage_Level : Inport  Port=3
  Control_Surface_Cmd : Inport  Port=4
  Add : Sum
  Constant2 : Constant  Value=FCC_PIX_Data.Servo.PWM.Pulswidth_cmd_middle_pos_ms
  Constant6 : Constant  Value=FCC_PIX_Data.Servo.PWM.Pulswidth_cmd_max_ms-FCC_PIX_Data.Servo.PWM.Pulswidth_cmd_middle_pos_ms
  Divide : Product  Inputs=*/
  Mux : Mux  Inputs=3
  Product : Product
  Saturation : Saturate  UpperLimit=FCC_PIX_Data.Servo.PWM.Pulswidth_cmd_max_ms  LowerLimit=FCC_PIX_Data.Servo.PWM.Pulswidth_cmd_min_ms
  Servo_Cmd_PWM : Outport  VectorParamsAs1DForOutWhenUnconnected=off
  wires:
  Mux/1 -> Servo_Cmd_PWM/1
  max_Control_Surface_Deflection/1 -> Divide/2
  periode/1 -> Mux/2  "periode_ms"
  Saturation/1 -> Mux/1  "pulse_width_ms"
  Constant6/1 -> Product/1
  Product/1 -> Add/2
  Control_Surface_Cmd/1 -> Divide/1
  Voltage_Level/1 -> Mux/3  "voltage_level_V"
  Add/1 -> Saturation/1
  Divide/1 -> Product/2
  Constant2/1 -> Add/1

== system Pix_FCC_flash/ExecutionCycle/ACTION/Servo_Cmd_PIX/Servo_3 ==
  max_Control_Surface_Deflection : Inport
  periode : Inport  Port=2
  Voltage_Level : Inport  Port=3
  Control_Surface_Cmd : Inport  Port=4
  Add : Sum
  Constant2 : Constant  Value=FCC_PIX_Data.Servo.PWM.Pulswidth_cmd_middle_pos_ms
  Constant6 : Constant  Value=FCC_PIX_Data.Servo.PWM.Pulswidth_cmd_max_ms-FCC_PIX_Data.Servo.PWM.Pulswidth_cmd_middle_pos_ms
  Divide : Product  Inputs=*/
  Mux : Mux  Inputs=3
  Product : Product
  Saturation : Saturate  UpperLimit=FCC_PIX_Data.Servo.PWM.Pulswidth_cmd_max_ms  LowerLimit=FCC_PIX_Data.Servo.PWM.Pulswidth_cmd_min_ms
  Servo_Cmd_PWM : Outport  VectorParamsAs1DForOutWhenUnconnected=off
  wires:
  Mux/1 -> Servo_Cmd_PWM/1
  max_Control_Surface_Deflection/1 -> Divide/2
  periode/1 -> Mux/2  "periode_ms"
  Saturation/1 -> Mux/1  "pulse_width_ms"
  Constant6/1 -> Product/1
  Product/1 -> Add/2
  Control_Surface_Cmd/1 -> Divide/1
  Voltage_Level/1 -> Mux/3  "voltage_level_V"
  Add/1 -> Saturation/1
  Divide/1 -> Product/2
  Constant2/1 -> Add/1

== system Pix_FCC_flash/ExecutionCycle/ACTION/Servo_Cmd_PIX/Servo_4 ==
  max_Control_Surface_Deflection : Inport
  periode : Inport  Port=2
  Voltage_Level : Inport  Port=3
  Control_Surface_Cmd : Inport  Port=4
  Add : Sum
  Constant2 : Constant  Value=FCC_PIX_Data.Servo.PWM.Pulswidth_cmd_middle_pos_ms
  Constant6 : Constant  Value=FCC_PIX_Data.Servo.PWM.Pulswidth_cmd_max_ms-FCC_PIX_Data.Servo.PWM.Pulswidth_cmd_middle_pos_ms
  Divide : Product  Inputs=*/
  Mux : Mux  Inputs=3
  Product : Product
  Saturation : Saturate  UpperLimit=FCC_PIX_Data.Servo.PWM.Pulswidth_cmd_max_ms  LowerLimit=FCC_PIX_Data.Servo.PWM.Pulswidth_cmd_min_ms
  Servo_Cmd_PWM : Outport  VectorParamsAs1DForOutWhenUnconnected=off
  wires:
  Mux/1 -> Servo_Cmd_PWM/1
  max_Control_Surface_Deflection/1 -> Divide/2
  periode/1 -> Mux/2  "periode_ms"
  Saturation/1 -> Mux/1  "pulse_width_ms"
  Constant6/1 -> Product/1
  Product/1 -> Add/2
  Control_Surface_Cmd/1 -> Divide/1
  Voltage_Level/1 -> Mux/3  "voltage_level_V"
  Add/1 -> Saturation/1
  Divide/1 -> Product/2
  Constant2/1 -> Add/1

== system Pix_FCC_flash/ExecutionCycle/OUTPUT/serial send/Send Data ==
  data : Inport
  function : TriggerPort  TriggerType=function-call  VariantControl=Variant
  Constant : Constant  Value=[1 2 3]'
  Serial Transmit : px4lib/Serial Transmit  SCIModule=/dev/ttyS6
      settings: SourceProductName=Embedded Coder Support Package for PX4 Autopilots  SourceProductBaseCode=PX4AUTOPILOTS
  Terminator : Terminator
  wires:
  Constant/1 -> Serial Transmit/1
  data/1 -> Terminator/1

== system Pix_FCC_flash/ExecutionCycle/OUTPUT/serial send/Send Header ==
  function : TriggerPort  TriggerType=function-call  VariantControl=Variant
  Header : Constant  Value=[5 5]  OutDataTypeStr=uint8  SampleTime=-1
  Serial Transmit : px4lib/Serial Transmit  SCIModule=/dev/ttyS6
      settings: SourceProductName=Embedded Coder Support Package for PX4 Autopilots  SourceProductBaseCode=PX4AUTOPILOTS
  wires:
  Header/1 -> Serial Transmit/1

== system Pix_FCC_flash/ExecutionCycle/OUTPUT/serial send/Send Terminator ==
  function : TriggerPort  TriggerType=function-call  VariantControl=Variant
  Header : Constant  Value=[5 5]  OutDataTypeStr=uint8  SampleTime=-1
  Serial Transmit : px4lib/Serial Transmit  SCIModule=/dev/ttyS6
      settings: SourceProductName=Embedded Coder Support Package for PX4 Autopilots  SourceProductBaseCode=PX4AUTOPILOTS
  wires:
  Header/1 -> Serial Transmit/1

== system Pix_FCC_flash/ExecutionCycle/OUTPUT/serial send/Send WhiteNoise Beginning ==
  function : TriggerPort  TriggerType=function-call  VariantControl=Variant
  Header : Constant  Value=[0 0 0 0 0]  OutDataTypeStr=uint8  SampleTime=-1
  Serial Transmit : px4lib/Serial Transmit  SCIModule=/dev/ttyS6
      settings: SourceProductName=Embedded Coder Support Package for PX4 Autopilots  SourceProductBaseCode=PX4AUTOPILOTS
  wires:
  Header/1 -> Serial Transmit/1

== system Pix_FCC_flash/ExecutionCycle/OUTPUT/serial send/Send WhiteNoise End ==
  function : TriggerPort  TriggerType=function-call  VariantControl=Variant
  Header : Constant  Value=[0 0 0 0 0]  OutDataTypeStr=uint8  SampleTime=-1
  Serial Transmit : px4lib/Serial Transmit  SCIModule=/dev/ttyS6
      settings: SourceProductName=Embedded Coder Support Package for PX4 Autopilots  SourceProductBaseCode=PX4AUTOPILOTS
  wires:
  Header/1 -> Serial Transmit/1

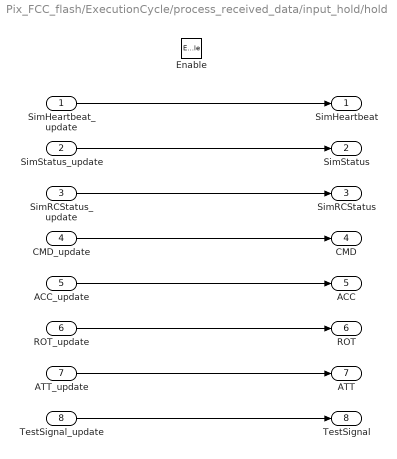
== system Pix_FCC_flash/ExecutionCycle/process_received_data/input_hold/hold ==
  SimHeartbeat_update : Inport
  SimStatus_update : Inport  Port=2
  SimRCStatus_update : Inport  Port=3
  CMD_update : Inport  Port=4
  ACC_update : Inport  Port=5
  ROT_update : Inport  Port=6
  ATT_update : Inport  Port=7
  TestSignal_update : Inport  Port=8
  Enable : EnablePort
  SimHeartbeat : Outport  VectorParamsAs1DForOutWhenUnconnected=off
  SimStatus : Outport  Port=2  VectorParamsAs1DForOutWhenUnconnected=off
  SimRCStatus : Outport  Port=3  VectorParamsAs1DForOutWhenUnconnected=off
  CMD : Outport  Port=4  VectorParamsAs1DForOutWhenUnconnected=off
  ACC : Outport  Port=5  VectorParamsAs1DForOutWhenUnconnected=off
  ROT : Outport  Port=6  VectorParamsAs1DForOutWhenUnconnected=off
  ATT : Outport  Port=7  VectorParamsAs1DForOutWhenUnconnected=off
  TestSignal : Outport  Port=8  VectorParamsAs1DForOutWhenUnconnected=off
  wires:
  SimHeartbeat_update/1 -> SimHeartbeat/1
  SimStatus_update/1 -> SimStatus/1
  SimRCStatus_update/1 -> SimRCStatus/1
  CMD_update/1 -> CMD/1
  ACC_update/1 -> ACC/1
  ROT_update/1 -> ROT/1
  ATT_update/1 -> ATT/1
  TestSignal_update/1 -> TestSignal/1

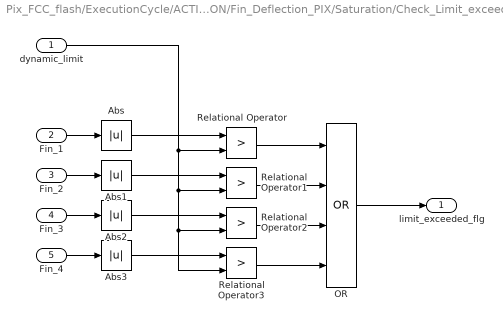
== system Pix_FCC_flash/ExecutionCycle/ACTION/Fin_Deflection_PIX/Saturation/Check_Limit_exceeding ==
  dynamic_limit : Inport
  Fin_1 : Inport  Port=2
  Fin_2 : Inport  Port=3
  Fin_3 : Inport  Port=4
  Fin_4 : Inport  Port=5
  Abs{,1..3} (4 alike) : Abs
  OR : Logic  Operator=OR  Inputs=4  IconShape=distinctive  AllPortsSameDT=off  OutDataTypeStr=boolean
  Relational Operator{,1..3} (4 alike) : RelationalOperator  Operator=>  OutDataTypeStr=boolean  RndMeth=Simplest
  limit_exceeded_flg : Outport  VectorParamsAs1DForOutWhenUnconnected=off
  wires:
  dynamic_limit/1 -> Relational Operator1/2, Relational Operator2/2, Relational Operator3/2, Relational Operator/2
  Abs3/1 -> Relational Operator3/1
  Abs2/1 -> Relational Operator2/1
  Abs1/1 -> Relational Operator1/1
  Abs/1 -> Relational Operator/1
  Relational Operator3/1 -> OR/4
  Relational Operator2/1 -> OR/3
  Relational Operator1/1 -> OR/2
  Relational Operator/1 -> OR/1
  Fin_1/1 -> Abs/1
  Fin_2/1 -> Abs1/1
  Fin_3/1 -> Abs2/1
  Fin_4/1 -> Abs3/1
  OR/1 -> limit_exceeded_flg/1

== system Pix_FCC_flash/ExecutionCycle/ACTION/Fin_Deflection_PIX/Saturation/Pass ==
  Fin_1_Cmd_rad : Inport
  Fin_2_Cmd_rad : Inport  Port=2
  Fin_3_Cmd_rad : Inport  Port=3
  Fin_4_Cmd_rad : Inport  Port=4
  Enable : EnablePort
  Fin_1_Cmd_Sat_rad : Outport  VectorParamsAs1DForOutWhenUnconnected=off
  Fin_2_Cmd_Sat_rad : Outport  Port=2  VectorParamsAs1DForOutWhenUnconnected=off
  Fin_3_Cmd_Sat_rad : Outport  Port=3  VectorParamsAs1DForOutWhenUnconnected=off
  Fin_4_Cmd_Sat_rad : Outport  Port=4  VectorParamsAs1DForOutWhenUnconnected=off
  wires:
  Fin_3_Cmd_rad/1 -> Fin_3_Cmd_Sat_rad/1  "Fin_3_Cmd_rad"
  Fin_4_Cmd_rad/1 -> Fin_4_Cmd_Sat_rad/1  "Fin_4_Cmd_rad"
  Fin_1_Cmd_rad/1 -> Fin_1_Cmd_Sat_rad/1  "Fin_1_Cmd_rad"
  Fin_2_Cmd_rad/1 -> Fin_2_Cmd_Sat_rad/1  "Fin_2_Cmd_rad"

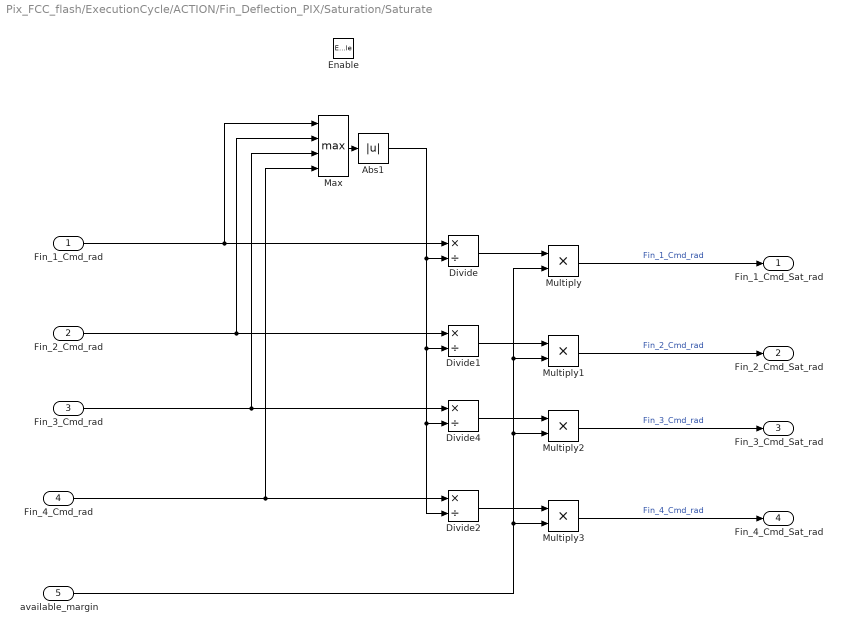
== system Pix_FCC_flash/ExecutionCycle/ACTION/Fin_Deflection_PIX/Saturation/Saturate ==
  Fin_1_Cmd_rad : Inport
  Fin_2_Cmd_rad : Inport  Port=2
  Fin_3_Cmd_rad : Inport  Port=3
  Fin_4_Cmd_rad : Inport  Port=4
  available_margin : Inport  Port=5
  Enable : EnablePort
  Abs1 : Abs
  Divide{,1..2,4} (4 alike) : Product  Inputs=*/
  Max : MinMax  Function=max  Inputs=4
  Multiply{,1..3} (4 alike) : Product
  Fin_1_Cmd_Sat_rad : Outport  VectorParamsAs1DForOutWhenUnconnected=off
  Fin_2_Cmd_Sat_rad : Outport  Port=2  VectorParamsAs1DForOutWhenUnconnected=off
  Fin_3_Cmd_Sat_rad : Outport  Port=3  VectorParamsAs1DForOutWhenUnconnected=off
  Fin_4_Cmd_Sat_rad : Outport  Port=4  VectorParamsAs1DForOutWhenUnconnected=off
  wires:
  available_margin/1 -> Multiply3/2, Multiply2/2, Multiply1/2, Multiply/2
  Multiply2/1 -> Fin_3_Cmd_Sat_rad/1  "Fin_3_Cmd_rad"
  Multiply3/1 -> Fin_4_Cmd_Sat_rad/1  "Fin_4_Cmd_rad"
  Multiply/1 -> Fin_1_Cmd_Sat_rad/1  "Fin_1_Cmd_rad"
  Divide4/1 -> Multiply2/1
  Max/1 -> Abs1/1
  Fin_3_Cmd_rad/1 -> Divide4/1, Max/3
  Fin_4_Cmd_rad/1 -> Divide2/1, Max/4
  Fin_2_Cmd_rad/1 -> Divide1/1, Max/2
  Multiply1/1 -> Fin_2_Cmd_Sat_rad/1  "Fin_2_Cmd_rad"
  Abs1/1 -> Divide/2, Divide1/2, Divide4/2, Divide2/2
  Divide2/1 -> Multiply3/1
  Divide1/1 -> Multiply1/1
  Divide/1 -> Multiply/1
  Fin_1_Cmd_rad/1 -> Divide/1, Max/1

== matlab function Pix_FCC_flash/ExecutionCycle/process_received_data/input_hold/ExtractMessage ==
  data: data input uint8 size=[128 1]; message output uint8 size=[1 56]; packetfound output
function [message,packetfound] = ExtractMessage(data)
    
    %specify size and type of input and output data in data manager!!
    
    data = data';
    expected_message_length = 56; % specify!!
    expected_header = [7 7];      % specify!!
    expected_header_length = length(expected_header);
    expected_packet_length = expected_message_length + expected_header_length;
    
    packet = uint8(zeros(1,expected_message_length));
    packetfound = false;
    
    %% locate packet in data
    
    % First, find possible header start locations; i.e., match the first element in the
    % header.
    start = find(data==expected_header(1));
    
    % Next remove start values that are too close to the end to possibly match
    % the header.
    endVals = start+expected_header_length-1;
    start(endVals>length(data)) = [];
    
    % Next, loop over elements of header, usually much shorter than length of
    % array, to check which possible header start locations are valid still.
    for pattval = 2:expected_header_length
        % check viable locations in array
        locs = expected_header(pattval) == data(start+pattval-1);
        % delete false ones from indices
        start(~locs) = [];
    end
    
    %Packet = Data - Header
    if ~isempty(start)
        for i = 1:(length(start)-1)
            %Verify if the size of data between 2 consecutive header start
            %indices is equal to the expectedPacketSize
            if isequal(start(i+1)-start(i),expected_packet_length)
            
                %Extract the packet by stripping the header from the data
                packet = data(start(i)+expected_header_length:start(i+1)-1);
                if ~isequal(length(packet),(expected_packet_length-expected_header_length))
                    error('ERROR:Wrong packet size');
                end
            
                %Once a valid packet is found, exit the for loop
                packetfound = true;
                break;
            else
                continue
            end
        end
    else
        packetfound = false;
    end
    
    
    
    %% extract message
    
    message = uint8(packet);
    
    
    
    
    
    
end

== matlab function Pix_FCC_flash/ExecutionCycle/OUTPUT/serial send/MessageAssembly ==
  data: SendingMode input double size=1; MessageAddition output single size=1; PixHeartbeat input uint16 size=1; PixStatus input uint8 size=1; RCStatus input uint8 size=1
function MessageAddition = MessageAssembly(SendingMode, PixHeartbeat, PixStatus, RCStatus)
    
    
    %specify size and type of input and output data in data manager!!
    
    if SendingMode == 1
        
        package = [typecast(uint16(PixHeartbeat),'uint8') PixStatus RCStatus];
        
        MessageAddition = typecast(uint8(package),'single');
        
    else
        
        MessageAddition = single(0);
        
    end
    
    
end
